simulink model "simpleCylinder1"  (Simulink 6.5)
settings: Solver=ode4  StartTime=0.0  StopTime=inf  FixedStep=0.001  RelTol=1e-3
undefined symbols (not defined in the file or in its folder): x
libraries: dsparch4 x5, xpclib x4, simulink x4
settings Model: Creator=Administrator  LastModifiedBy=PC  BufferReuse=off
settings ConfigSet: SimulationMode=external
settings OptimizationCC: BlockReduction=off  OptimizeBlockIOStorage=off  BufferReuse=off  ExpressionFolding=off  LocalBlockOutputs=off
settings RTWCC: SystemTargetFile=xpctarget.tlc  TemplateMakefile=xpc_default_tmf  Description=xPC Target  ProcessScript=xpctarget_make_rtw_hook
settings xpcTargetCC: TargetFcnLib=ansi_tfl_tmw.mat  GenFloatMathFcnCalls=ANSI_C  ExtModeInterfaceLevel=Level2 - Open

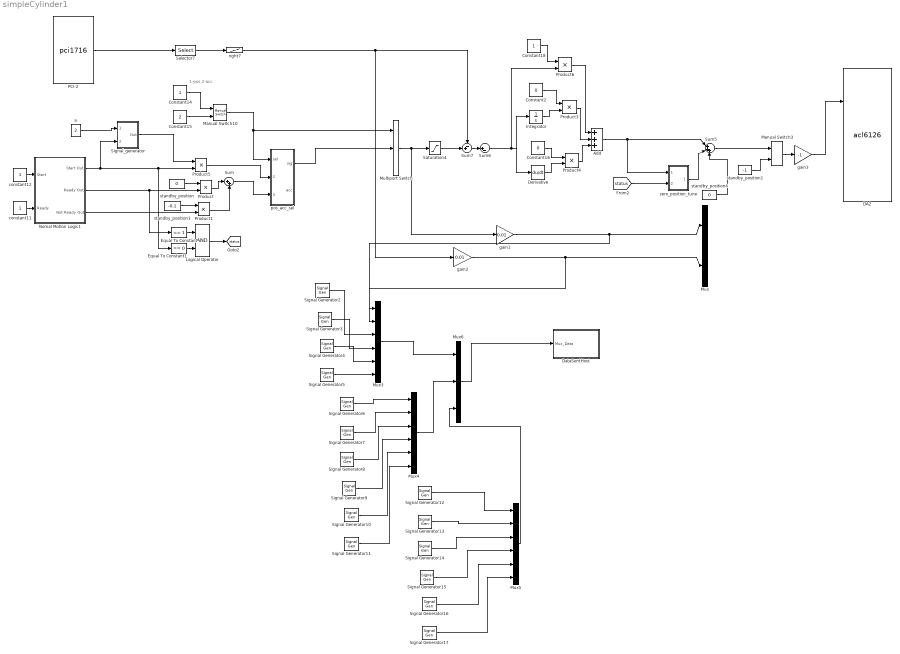
== system simpleCylinder1 ==
  note: 1-pos
      | 2-acc
  Add : Sum  Inputs=+++  OutScaling=2^-10
  Constant14 : Constant  Value=1  OutDataType=fixdt(1,16,0)  ConRadixGroup=Use specified scaling  OutScaling=[]  SampleTime=inf  FramePeriod=inf
  Constant15 : Constant  Value=2  OutDataType=fixdt(1,16,0)  ConRadixGroup=Use specified scaling  OutScaling=[]  SampleTime=inf  FramePeriod=inf
  Constant16 : Constant  Value=0  OutDataType=fixdt(1,16,0)  ConRadixGroup=Use specified scaling  OutScaling=[]  SampleTime=inf  FramePeriod=inf
  Constant18 : Constant  Value=1  OutDataType=fixdt(1,16,0)  ConRadixGroup=Use specified scaling  OutScaling=[]  SampleTime=inf  FramePeriod=inf
  Constant2 : Constant  Value=0  OutDataType=fixdt(1,16,0)  ConRadixGroup=Use specified scaling  OutScaling=[]  SampleTime=inf  FramePeriod=inf
  DA2 : S-Function  FunctionName=acl6126  Parameters=convBaseAddr,Range,[SampleTime SampleOffset]  mask(ACL-6126){sBaseAddr=0x2c0, Ranges=-10, sample=0.001}
      mask prompts: sBaseAddr "Base Address:"; sample "Sample Time:"
      mask help:
      | ACL-6126
      | HIT
      | Analog Output
      mask init:
      | convBaseAddr = 512;Range=10;SampleTime = 0.001; SampleOffset = 0;
      | sampleLength = length (sample);
      | if (sampleLength == 2)
      |   SampleTime = sample(1);
      |   SampleOffset = sample(2);
      | else
      |   SampleTime = sample(1);
      |   SampleOffset = 0;
      | end
      | 
      | sBaseAddr(find(sBaseAddr=='''')) = [];
      | index = findstr(lower(sBaseAddr),'0x');
      | if ~isempty(index) & index==1
      |   BaseAddr = sBaseAddr(3:end);
      |   baLength = length (BaseAddr);
      |   baseStringMember = [abs('0'):abs('9'),abs('a'):abs('f'),abs('A'):abs('F')];
      |   for i = 1:baLength
      |  %   if ~ismember(BaseAddr(i),baseStringMember)
      |  %     error ('Invalid character in hexadecimal string');
      |  %   end
      |   end
      |   convBaseAddr = hex2dec(BaseAddr);
      | else
      |   convBaseAddr = str2num(BaseAddr);
      |   end
      |  Range=Ranges;
      mask Help: helpview([docroot '/toolbox/xpc/pt_io_block_reference.html#xpcioref'])
      mask Display:
      | disp('ACL-6126\ncumt\nAnalog Output');
      | port_label('input',1 , '1');
      | port_label('input',2 , '2');
      | port_label('input',3 , '3');
      | port_label('input',4 , '4');
      | port_label('input',5, '5');
      | port_label('input',6 , '6');
  DataSentHost : Subsystem
  Derivative : Derivative
  Equal To Constant : simulink/Logic and Bit Operations/Compare To Constant  SystemSampleTime=-1  relop===  const=1  LogicOutDataTypeMode=uint8  ZeroCross=off
  Equal To Constant1 : simulink/Logic and Bit Operations/Compare To Constant  SystemSampleTime=-1  relop===  const=0  LogicOutDataTypeMode=uint8  ZeroCross=off
  Integrator : Integrator
  Logical Operator : Logic  AllPortsSameDT=off
  Manual Switch10 : simulink/Signal Routing/Manual Switch  SystemSampleTime=-1  sw=1  action=0
  Manual Switch3 : simulink/Signal Routing/Manual Switch  SystemSampleTime=-1  sw=0  action=0
  Multiport Switch : MultiPortSwitch  Inputs=2  SaturateOnIntegerOverflow=on
  Mux : Mux  Inputs=2
  Mux3 : Mux  Inputs=6
  Mux4 : Mux  Inputs=6
  Mux5 : Mux  Inputs=6
  Mux6 : Mux  Inputs=3
  Nomal Motion Logic1 : Subsystem  AncestorBlock=control_logic_lib/Control Logic(Stateflow Chart)
  PCI-2 : S-Function  FunctionName=pci1716  Parameters=[SampleTime SampleOffset], SLOT  mask(hitad3){Sample=0.001, SLOT=-1}
      mask prompts: Sample "Sample Time:"
      mask help:
      | PCi1716
      | A/D Card
      | Developed by ZhaoJinsong
      | 2012.06.02
      mask init:
      | SampleTime = 0.001; SampleOffset=0;
      mask Help: helpview([docroot '/toolbox/xpc/pt_io_block_reference.html#xpcioref'])
      mask Display:
      | disp('PCI1716  ');
      | 
      | port_label('output',1 , 'OUT');
  Product : Product  OutDataType=fixdt(1,16,0)  OutScaling=[]  SaturateOnIntegerOverflow=on
  Product1 : Product  OutDataType=fixdt(1,16,0)  OutScaling=[]  SaturateOnIntegerOverflow=on
  Product3 : Product  RndMeth=Zero
  Product4 : Product  RndMeth=Zero
  Product5 : Product  OutDataType=fixdt(1,16,0)  OutScaling=[]  SaturateOnIntegerOverflow=on
  Product6 : Product  RndMeth=Zero
  Saturation4 : Saturate  UpperLimit=10  LowerLimit=-10
  Selector7 : Selector  InputType=Vector  ElementSrc=Internal  Elements=2  RowSrc=Internal  Rows=1  ColumnSrc=Internal  Columns=1  IndexIsStartValue=off
  Signal Generator10 : SignalGenerator  Amplitude=11  Frequency=10
  Signal Generator11 : SignalGenerator  Amplitude=12  Frequency=10
  Signal Generator12 : SignalGenerator  Amplitude=13  Frequency=10
  Signal Generator13 : SignalGenerator  Amplitude=14  Frequency=10
  Signal Generator14 : SignalGenerator  Amplitude=15  Frequency=10
  Signal Generator15 : SignalGenerator  Amplitude=16  Frequency=10
  Signal Generator16 : SignalGenerator  Amplitude=17  Frequency=10
  Signal Generator17 : SignalGenerator  Amplitude=18  Frequency=10
  Signal Generator2 : SignalGenerator  Amplitude=3  Frequency=10
  Signal Generator3 : SignalGenerator  Amplitude=4  Frequency=10
  Signal Generator4 : SignalGenerator  Amplitude=5  Frequency=10
  Signal Generator5 : SignalGenerator  Amplitude=6  Frequency=10
  Signal Generator6 : SignalGenerator  Amplitude=7  Frequency=10
  Signal Generator7 : SignalGenerator  Amplitude=8  Frequency=10
  Signal Generator8 : SignalGenerator  Amplitude=9  Frequency=10
  Signal Generator9 : SignalGenerator  Amplitude=10  Frequency=10
  Signal_generator : Subsystem
  Sum : Sum  Inputs=|++  OutDataType=fixdt(1,16,0)  OutScaling=[]  SaturateOnIntegerOverflow=on
  Sum5 : Sum  Inputs=|+++  OutDataType=fixdt(1,16,0)  OutScaling=[]  SaturateOnIntegerOverflow=on
  Sum6 : Sum  Inputs=|+-  OutDataType=fixdt(1,16,0)  OutScaling=[]  SaturateOnIntegerOverflow=on
  Sum7 : Sum  Inputs=-+|  OutDataType=fixdt(1,16,0)  OutScaling=[]  SaturateOnIntegerOverflow=on
  a : Constant  Value=2  OutDataType=fixdt(1,16,0)  ConRadixGroup=Use specified scaling  OutScaling=[]  SampleTime=inf  FramePeriod=inf
  constant11 : Constant  Value=1  OutDataType=sfix(16)  ConRadixGroup=Use specified scaling  OutScaling=2^0  SampleTime=inf  FramePeriod=inf
      settings: OpenFcn=|
      | if get_param(gcb,'value')=='1',
      | set_param(gcb,'value','0');
      | else
      | set_param(gcb,'value','1');end
  constant12 : Constant  Value=1  OutDataType=sfix(16)  ConRadixGroup=Use specified scaling  OutScaling=2^0  SampleTime=inf  FramePeriod=inf
      settings: OpenFcn=|
      | if get_param(gcb,'value')=='1',
      | set_param(gcb,'value','0');
      | else
      | set_param(gcb,'value','1');end
  gain1 : Gain  Gain=0.01  ParameterDataType=fixdt(1,16,0)  ParameterScaling=[]  OutDataType=fixdt(1,16,0)  OutScaling=[]  SaturateOnIntegerOverflow=on
  gain2 : Gain  Gain=0.01  ParameterDataType=fixdt(1,16,0)  ParameterScaling=[]  OutDataType=fixdt(1,16,0)  OutScaling=[]  SaturateOnIntegerOverflow=on
  gain3 : Gain  Gain=-1  ParameterDataType=fixdt(1,16,0)  ParameterScaling=[]  OutDataType=fixdt(1,16,0)  OutScaling=[]  SaturateOnIntegerOverflow=on
  pos_acc_sel : Subsystem
  right7 : Lookup  InputValues=[-0.28 9.725]  OutputValues=[-10 10]  LookUpMeth=Interpolation-Extrapolation  OutDataType=fixdt(1,16,0)  OutScaling=[]  SaturateOnIntegerOverflow=on  SampleTime=-1  LUTDesignTableMode=Redesign Table  LUTDesignDataSource=Block Dialog  LUTDesignFunctionName=sqrt(x)  LUTDesignUseExistingBP=on  LUTDesignRelError=0.01  LUTDesignAbsError=1e-6  RndMeth=Floor
      settings: LockScale=off
  standby_position : Constant  Value=0  OutDataType=fixdt(1,16,0)  ConRadixGroup=Use specified scaling  OutScaling=[]  SampleTime=inf  FramePeriod=inf
  standby_position1 : Constant  Value=-1  OutDataType=fixdt(1,16,0)  ConRadixGroup=Use specified scaling  OutScaling=[]  SampleTime=inf  FramePeriod=inf
  standby_position3 : Constant  Value=-0.1  OutDataType=fixdt(1,16,0)  ConRadixGroup=Use specified scaling  OutScaling=[]  SampleTime=inf  FramePeriod=inf
  standby_position4 : Constant  Value=0  OutDataType=fixdt(1,16,0)  ConRadixGroup=Use specified scaling  OutScaling=[]  SampleTime=inf  FramePeriod=inf
  zero_position_tune : Subsystem
  tag scope: status=global
  wires:
  standby_position1/1 -> Manual Switch3/2
  Manual Switch3/1 -> gain3/1
  Mux5/1 -> Mux6/3
  Mux4/1 -> Mux6/2
  Signal Generator12/1 -> Mux5/1
  Signal Generator13/1 -> Mux5/2
  Signal Generator14/1 -> Mux5/3
  Signal Generator15/1 -> Mux5/4
  Signal Generator16/1 -> Mux5/5
  Signal Generator17/1 -> Mux5/6
  Signal Generator6/1 -> Mux4/1
  Signal Generator7/1 -> Mux4/2
  Signal Generator8/1 -> Mux4/3
  Signal Generator9/1 -> Mux4/4
  Signal Generator10/1 -> Mux4/5
  Signal Generator11/1 -> Mux4/6
  Signal Generator5/1 -> Mux3/6
  Sum5/1 -> Manual Switch3/1
  standby_position4/1 -> Sum5/3
  Sum6/1 -> Product6/2, Integrator/1, Derivative/1
  Sum7/1 -> Sum6/1
  Multiport Switch/1 -> gain1/1, Saturation4/1
  pos_acc_sel/1(sig) -> Multiport Switch/2
  Saturation4/1 -> Sum7/2
  [status] -> zero_position_tune/2(status)
  zero_position_tune/1(Out) -> Sum5/2
  Constant2/1 -> Product3/1
  Integrator/1 -> Product3/2
  Constant16/1 -> Product4/1
  Derivative/1 -> Product4/2
  Constant18/1 -> Product6/1
  Product6/1 -> Add/1
  Product3/1 -> Add/2
  Product4/1 -> Add/3
  Add/1 -> Sum5/1, zero_position_tune/1(error_in)
  gain1/1 -> Mux/1, Mux3/1
  gain2/1 -> Mux/2, Mux3/2
  Mux6/1 -> DataSentHost/1(Mux_Data)
  Mux3/1 -> Mux6/1
  Signal Generator2/1 -> Mux3/3
  Signal Generator3/1 -> Mux3/4
  Signal Generator4/1 -> Mux3/5
  PCI-2/1 -> Selector7/1
  Selector7/1 -> right7/1
  right7/1 -> Sum7/1, gain2/1
  constant12/1 -> Nomal Motion Logic1/1(Start)
  Nomal Motion Logic1/2(Ready Out) -> Product/2, Equal To Constant/1
  standby_position/1 -> Product/1
  Product/1 -> Sum/1
  Sum/1 -> pos_acc_sel/3(ini_pos)
  Nomal Motion Logic1/1(Start Out) -> Product5/2, Equal To Constant1/1, Signal_generator/2(start)
  Product5/1 -> pos_acc_sel/2(sig_in)
  standby_position3/1 -> Product1/1
  Product1/1 -> Sum/2
  Manual Switch10/1 -> Multiport Switch/1, pos_acc_sel/1(sel)
  Constant14/1 -> Manual Switch10/1
  Constant15/1 -> Manual Switch10/2
  Nomal Motion Logic1/3(Not Ready Out) -> Product1/2
  Equal To Constant/1 -> Logical Operator/1
  Equal To Constant1/1 -> Logical Operator/2
  Logical Operator/1 -> [status]
  constant11/1 -> Nomal Motion Logic1/2(Ready)
  Signal_generator/1(Out) -> Product5/1
  a/1 -> Signal_generator/1(sig_sel)
  gain3/1 -> DA2/2

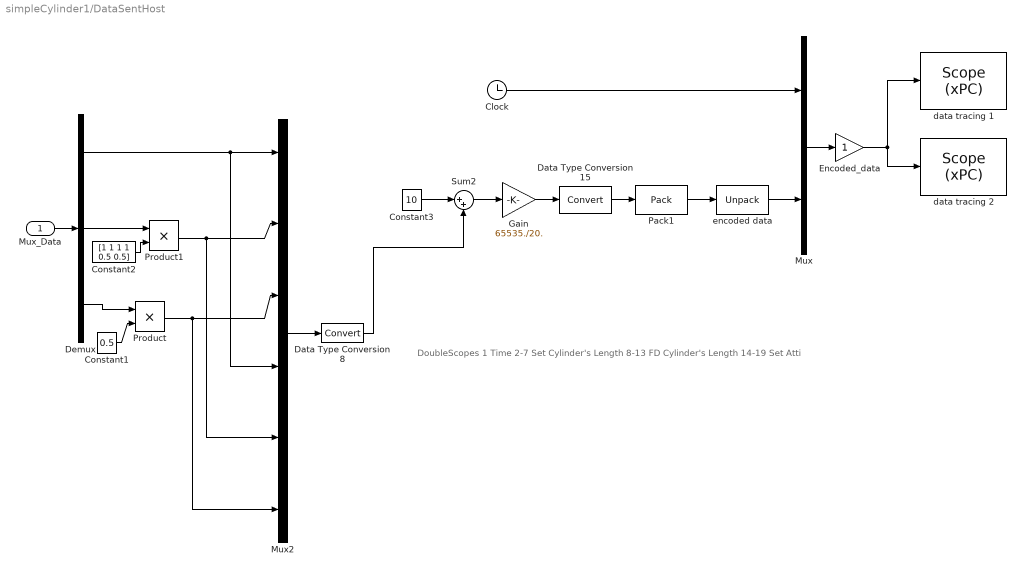
== system simpleCylinder1/DataSentHost ==
  note: DoubleScopes
      | 1          Time
      | 2-7       Set Cylinder's Length
      | 8-13     FD Cylinder's Length
      | 14-19   Set Atti
  Mux_Data : Inport
  Clock : Clock
      settings: Decimation=10
  Constant1 : Constant  Value=0.5  OutDataType=sfix(16)  ConRadixGroup=Use specified scaling  OutScaling=2^0  SampleTime=inf  FramePeriod=inf
  Constant2 : Constant  Value=[1 1 1 1 0.5 0.5]  OutDataType=sfix(16)  ConRadixGroup=Use specified scaling  OutScaling=2^0  SampleTime=inf  FramePeriod=inf
  Constant3 : Constant  Value=10  OutDataType=sfix(16)  ConRadixGroup=Use specified scaling  OutScaling=2^0  SampleTime=inf  FramePeriod=inf
  Data Type Conversion15 : DataTypeConversion  OutDataTypeMode=uint16  SaturateOnIntegerOverflow=on  RndMeth=Zero
  Data Type Conversion8 : DataTypeConversion  OutDataTypeMode=double  SaturateOnIntegerOverflow=on  RndMeth=Zero
  Demux : Demux  Outputs=3
  Encoded_data : Gain
  Gain : Gain  Gain=65535./20.  RndMeth=Nearest  SaturateOnIntegerOverflow=on
  Mux : Mux  Inputs=2
  Mux2 : Mux  Inputs=6
  Pack1 : xpclib/UDP/Pack  datatypes={'uint16'}  byteAlign=1
  Product : Product  RndMeth=Zero
  Product1 : Product  RndMeth=Zero
  Sum2 : Sum  Inputs=|++  SaturateOnIntegerOverflow=on
  data tracing 1 : xpclib/Misc./Scope (xPC)   SystemSampleTime=-1  scopeno=5  scopetype=Host  autostart=off  viewmode=Graphical redraw  formatstr='%15.6f'  grid=on  ylimits=[0,0]  nosamples=500  noprepostsamples=0  interleave=1  triggermode=Scope triggering  triggersignal=1  triggerlevel=0.0  triggerslope=Either  triggerscope=5  triggersample=-1  filename=data.dat  mode=Lazy  writesize=512  autorestart=off
  data tracing 2 : xpclib/Misc./Scope (xPC)   SystemSampleTime=-1  scopeno=4  scopetype=Host  autostart=off  viewmode=Graphical redraw  formatstr='%15.6f'  grid=on  ylimits=[0,0]  nosamples=500  noprepostsamples=0  interleave=1  triggermode=Scope triggering  triggersignal=1  triggerlevel=0.0  triggerslope=Either  triggerscope=4  triggersample=-1  filename=data.dat  mode=Lazy  writesize=512  autorestart=off
  encoded data : xpclib/UDP/Unpack  dimensions={[9]}  datatypes={'double'}  byteAlign=1
  wires:
  Constant2/1 -> Product1/2
  Product1/1 -> Mux2/5, Mux2/2
  Demux/2 -> Product1/1
  Product/1 -> Mux2/6, Mux2/3
  Constant1/1 -> Product/2
  Demux/3 -> Product/1
  Encoded_data/1 -> data tracing 2/1, data tracing 1/1
  Mux/1 -> Encoded_data/1
  Demux/1 -> Mux2/4, Mux2/1
  Mux_Data/1 -> Demux/1
  Clock/1 -> Mux/1
  Constant3/1 -> Sum2/1
  Sum2/1 -> Gain/1
  Pack1/1 -> encoded data/1
  Gain/1 -> Data Type Conversion15/1
  Data Type Conversion15/1 -> Pack1/1
  encoded data/1 -> Mux/2
  Mux2/1 -> Data Type Conversion8/1
  Data Type Conversion8/1 -> Sum2/2

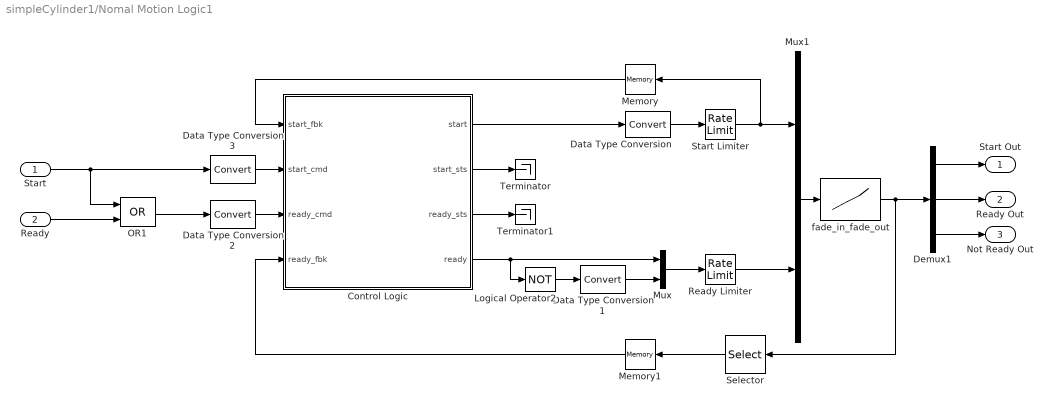
== system simpleCylinder1/Nomal Motion Logic1 ==
  Start : Inport
  Ready : Inport  Port=2
  Control Logic : Stateflow chart
  Data Type Conversion{,1..3} (4 alike) : DataTypeConversion  OutDataTypeMode=double  SaturateOnIntegerOverflow=on  RndMeth=Zero
  Demux1 : Demux  Outputs=3
  Logical Operator2 : Logic  Operator=NOT  Inputs=3  AllPortsSameDT=off
  Memory : Memory  Orientation=left
  Memory1 : Memory  Orientation=left
  Mux : Mux  Inputs=2
  Mux1 : Mux  Inputs=2
  OR1 : Logic  Operator=OR  AllPortsSameDT=off
  Ready Limiter : RateLimiter  RisingSlewLimit=1/5  FallingSlewLimit=-1/5
  Selector : Selector  Orientation=left  InputType=Vector  ElementSrc=Internal  Elements=[2]  RowSrc=Internal  Rows=[2]  ColumnSrc=Internal  Columns=1  InputPortWidth=3  IndexIsStartValue=off  OutputPortSize=[(-2)]
  Start Limiter : RateLimiter  RisingSlewLimit=1/3  FallingSlewLimit=-1/3
  Terminator : Terminator
  Terminator1 : Terminator
  fade_in_fade_out : Lookup  InputValues=[0:0.001:1]  OutputValues=(sin(([0:0.001:1]*2-1)*pi/2)+1)/2  LookUpMeth=Interpolation-Extrapolation  OutDataType=sfix(16)  OutScaling=2^0  SaturateOnIntegerOverflow=on  SampleTime=-1  LUTDesignTableMode=Redesign Table  LUTDesignDataSource=Block Dialog  LUTDesignFunctionName=sqrt(x)  LUTDesignUseExistingBP=on  LUTDesignRelError=0.01  LUTDesignAbsError=1e-6  RndMeth=Floor
      settings: LockScale=off
  Start Out : Outport
  Ready Out : Outport  Port=2
  Not Ready Out : Outport  Port=3
  wires:
  Ready/1 -> OR1/2
  Start/1 -> OR1/1, Data Type Conversion3/1
  Control Logic/3(ready_sts) -> Terminator1/1
  Control Logic/2(start_sts) -> Terminator/1
  OR1/1 -> Data Type Conversion2/1
  Data Type Conversion3/1 -> Control Logic/2(start_cmd)
  Demux1/3 -> Not Ready Out/1
  Demux1/1 -> Start Out/1
  Demux1/2 -> Ready Out/1
  Data Type Conversion/1 -> Start Limiter/1
  Start Limiter/1 -> Mux1/1, Memory/1
  Control Logic/1(start) -> Data Type Conversion/1
  Control Logic/4(ready) -> Logical Operator2/1, Mux/1
  Logical Operator2/1 -> Data Type Conversion1/1
  Mux/1 -> Ready Limiter/1
  Ready Limiter/1 -> Mux1/2
  Mux1/1 -> fade_in_fade_out/1
  fade_in_fade_out/1 -> Selector/1, Demux1/1
  Memory/1 -> Control Logic/1(start_fbk)
  Memory1/1 -> Control Logic/4(ready_fbk)
  Data Type Conversion1/1 -> Mux/2
  Data Type Conversion2/1 -> Control Logic/3(ready_cmd)
  Selector/1 -> Memory1/1

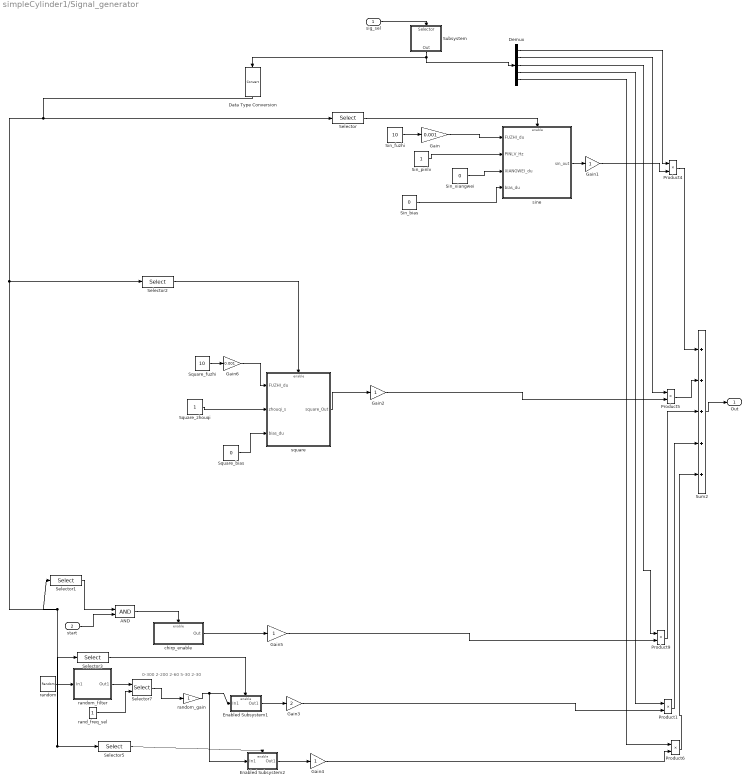
== system simpleCylinder1/Signal_generator ==
  note: 0-300
      | 2-200
      | 2-60
      | 5-30
      | 2-30
  sig_sel : Inport  OutDataType=fixdt(1,16,0)  OutScaling=[]
  start : Inport  Port=2  OutDataType=fixdt(1,16,0)  OutScaling=[]
  AND : Logic  AllPortsSameDT=off  OutDataTypeMode=Specify via dialog
  Data Type Conversion : DataTypeConversion  Orientation=down  OutDataTypeMode=boolean  OutDataType=fixdt(1,16,0)  OutScaling=[]  SaturateOnIntegerOverflow=on  RndMeth=Zero
  Demux : Demux  Outputs=5
  Enabled Subsystem1 : Subsystem  TreatAsAtomicUnit=on
  Enabled Subsystem2 : Subsystem  TreatAsAtomicUnit=on
  Gain : Gain  Gain=0.001
  Gain{1..2,4..5} (4 alike) : Gain  ParameterDataType=fixdt(1,16,0)  ParameterScaling=[]  OutDataType=fixdt(1,16,0)  OutScaling=[]  SaturateOnIntegerOverflow=on
  Gain3 : Gain  Gain=2  ParameterDataType=fixdt(1,16,0)  ParameterScaling=[]  OutDataType=fixdt(1,16,0)  OutScaling=[]  SaturateOnIntegerOverflow=on
  Gain6 : Gain  Gain=0.001
  Product{1,4..6,9} (5 alike) : Product  OutDataType=fixdt(1,16,0)  OutScaling=[]  SaturateOnIntegerOverflow=on
  Selector : Selector  InputType=Vector  ElementSrc=Internal  Elements=1  RowSrc=Internal  Rows=2  ColumnSrc=Internal  Columns=1  InputPortWidth=5  IndexIsStartValue=off  OutputPortSize=[(-2)]
  Selector1 : Selector  InputType=Vector  ElementSrc=Internal  Elements=3  RowSrc=Internal  Rows=4  ColumnSrc=Internal  Columns=1  InputPortWidth=5  IndexIsStartValue=off  OutputPortSize=[(-2)]
  Selector2 : Selector  InputType=Vector  ElementSrc=Internal  Elements=2  RowSrc=Internal  Rows=3  ColumnSrc=Internal  Columns=1  InputPortWidth=5  IndexIsStartValue=off  OutputPortSize=[(-2)]
  Selector3 : Selector  InputType=Vector  ElementSrc=Internal  Elements=4  RowSrc=Internal  Rows=5  ColumnSrc=Internal  Columns=1  InputPortWidth=5  IndexIsStartValue=off  OutputPortSize=[(-2)]
  Selector5 : Selector  InputType=Vector  ElementSrc=Internal  Elements=5  RowSrc=Internal  Rows=6  ColumnSrc=Internal  Columns=1  InputPortWidth=5  IndexIsStartValue=off  OutputPortSize=[(-2)]
  Selector7 : Selector  InputType=Vector  ElementSrc=External  Elements=[1 3]  RowSrc=External  Rows=[1 3]  ColumnSrc=Internal  Columns=1  InputPortWidth=5  IndexIsStartValue=off  OutputPortSize=[(-2)]
  Sin_bias : Constant  Value=0  OutDataType=sfix(16)  ConRadixGroup=Use specified scaling  OutScaling=2^0  SampleTime=inf  FramePeriod=inf
  Sin_fuzhi : Constant  Value=10  OutDataType=sfix(16)  ConRadixGroup=Use specified scaling  OutScaling=2^0  SampleTime=inf  FramePeriod=inf
  Sin_pinlv : Constant  Value=1  OutDataType=sfix(16)  ConRadixGroup=Use specified scaling  OutScaling=2^0  SampleTime=inf  FramePeriod=inf
  Sin_xiangwei : Constant  Value=0  OutDataType=sfix(16)  ConRadixGroup=Use specified scaling  OutScaling=2^0  SampleTime=inf  FramePeriod=inf
  Square_bias : Constant  Value=0  OutDataType=sfix(16)  ConRadixGroup=Use specified scaling  OutScaling=2^0  SampleTime=inf  FramePeriod=inf
  Square_fuzhi : Constant  Value=10  OutDataType=sfix(16)  ConRadixGroup=Use specified scaling  OutScaling=2^0  SampleTime=inf  FramePeriod=inf
  Square_zhouqi : Constant  Value=1  OutDataType=sfix(16)  ConRadixGroup=Use specified scaling  OutScaling=2^0  SampleTime=inf  FramePeriod=inf
  Subsystem : Subsystem  Orientation=down  mask{itnum=5}
      mask prompts: itnum "Signals Number"
  Sum2 : Sum  Inputs=+++++  OutDataType=fixdt(1,16,0)  OutScaling=[]  SaturateOnIntegerOverflow=on
  chirp_enable : Subsystem  TreatAsAtomicUnit=on
  rand_freq_sel : Constant  Value=1  OutDataType=fixdt(1,16,0)  ConRadixGroup=Use specified scaling  OutScaling=[]  SampleTime=inf  FramePeriod=inf
  random : UniformRandomNumber  SampleTime=0
  random_filter : Subsystem
  random_gain : Gain  ParameterDataType=fixdt(1,16,0)  ParameterScaling=[]  OutDataType=fixdt(1,16,0)  OutScaling=[]  SaturateOnIntegerOverflow=on
  sine : Subsystem
  square : Subsystem
  Out : Outport  OutDataType=fixdt(1,16,0)  OutScaling=[]
  wires:
  Product6/1 -> Sum2/5
  Demux/5 -> Product6/1
  Demux/4 -> Product1/1
  Gain5/1 -> Product9/2
  Demux/3 -> Product9/1
  Gain2/1 -> Product5/2
  Demux/2 -> Product5/1
  Product4/1 -> Sum2/1
  Demux/1 -> Product4/1
  Square_bias/1 -> square/3(bias_du)
  Sin_bias/1 -> sine/4(bias_du)
  Square_zhouqi/1 -> square/2(zhouqi_s)
  Square_fuzhi/1 -> Gain6/1
  Sin_xiangwei/1 -> sine/3(XIANGWEI_du)
  Sin_fuzhi/1 -> Gain/1
  Sin_pinlv/1 -> sine/2(PINLV_Hz)
  Selector/1 -> sine/Enable
  Gain3/1 -> Product1/2
  Product1/1 -> Sum2/4
  Selector7/1 -> random_gain/1
  Gain4/1 -> Product6/2
  Enabled Subsystem1/1(Out1) -> Gain3/1
  random_gain/1 -> Enabled Subsystem2/1(In1), Enabled Subsystem1/1(In1)
  Selector3/1 -> Enabled Subsystem1/Enable
  rand_freq_sel/1 -> Selector7/2
  random_filter/1(Out1) -> Selector7/1
  random/1 -> random_filter/1(In1)
  chirp_enable/1(Out) -> Gain5/1
  start/1 -> AND/2
  Selector1/1 -> AND/1
  AND/1 -> chirp_enable/Enable
  Enabled Subsystem2/1(Out1) -> Gain4/1
  sine/1(sin_out) -> Gain1/1
  Selector5/1 -> Enabled Subsystem2/Enable
  Selector2/1 -> square/Enable
  square/1(square_Out) -> Gain2/1
  Data Type Conversion/1 -> Selector/1, Selector3/1, Selector5/1, Selector1/1, Selector2/1
  Sum2/1 -> Out/1
  Product5/1 -> Sum2/2
  Product9/1 -> Sum2/3
  Subsystem/1(Out) -> Data Type Conversion/1, Demux/1
  sig_sel/1 -> Subsystem/1(Selector)
  Gain1/1 -> Product4/2
  Gain/1 -> sine/1(FUZHI_du)
  Gain6/1 -> square/1(FUZHI_du)

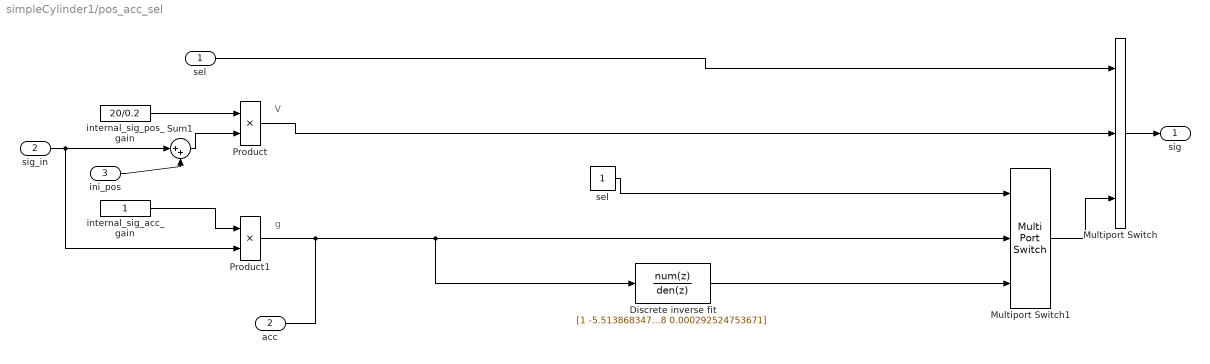
== system simpleCylinder1/pos_acc_sel ==
  note: g
  note: V
  sel : Inport  OutDataType=fixdt(1,16,0)  OutScaling=[]
  sig_in : Inport  Port=2  OutDataType=fixdt(1,16,0)  OutScaling=[]
  ini_pos : Inport  Port=3  OutDataType=fixdt(1,16,0)  OutScaling=[]
  Discrete inverse fit : DiscreteTransferFcn  Numerator=[1 -5.513868347662695 12.88491366007906 -16.323990002559352 11.821537968329908 -4.639485908156727 0.77101716333547]  Denominator=[0.013392688630559 -0.043519228995354 0.057088791124972 -0.038794303856191 0.015270049598488 -0.003637012524308 0.000292524753671]  SampleTime=0.001
  Multiport Switch : MultiPortSwitch  Inputs=2  SaturateOnIntegerOverflow=on
  Multiport Switch1 : MultiPortSwitch  Inputs=2  SaturateOnIntegerOverflow=on
  Product : Product  OutDataType=fixdt(1,16,0)  OutScaling=[]  SaturateOnIntegerOverflow=on
  Product1 : Product  OutDataType=fixdt(1,16,0)  OutScaling=[]  SaturateOnIntegerOverflow=on
  Sum1 : Sum  Inputs=|++  OutDataType=fixdt(1,16,0)  OutScaling=[]  SaturateOnIntegerOverflow=on
  internal_sig_acc_gain : Constant  Value=1  OutDataType=fixdt(1,16,0)  ConRadixGroup=Use specified scaling  OutScaling=[]  SampleTime=inf  FramePeriod=inf
  internal_sig_pos_gain : Constant  Value=20/0.2  OutDataType=fixdt(1,16,0)  ConRadixGroup=Use specified scaling  OutScaling=[]  SampleTime=inf  FramePeriod=inf
  "sel " : Constant  Value=1  OutDataType=fixdt(1,16,0)  ConRadixGroup=Use specified scaling  OutScaling=[]  SampleTime=inf  FramePeriod=inf
  sig : Outport  OutDataType=fixdt(1,16,0)  OutScaling=[]
  acc : Outport  Port=2  OutDataType=fixdt(1,16,0)  OutScaling=[]
  wires:
  internal_sig_acc_gain/1 -> Product1/1
  Product1/1 -> Discrete inverse fit/1, Multiport Switch1/2, acc/1
  internal_sig_pos_gain/1 -> Product/1
  Product/1 -> Multiport Switch/2
  Sum1/1 -> Product/2
  ini_pos/1 -> Sum1/2
  Multiport Switch/1 -> sig/1
  sel/1 -> Multiport Switch/1
  sig_in/1 -> Product1/2, Sum1/1
  Discrete inverse fit/1 -> Multiport Switch1/3
  "sel "/1 -> Multiport Switch1/1
  Multiport Switch1/1 -> Multiport Switch/3

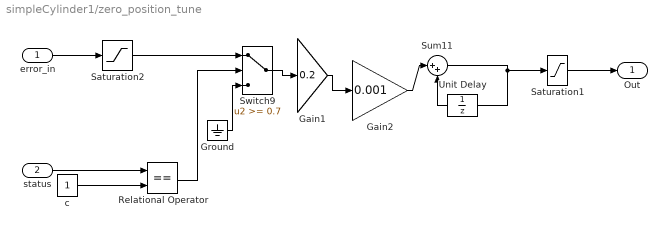
== system simpleCylinder1/zero_position_tune ==
  error_in : Inport  OutDataType=fixdt(1,16,0)  OutScaling=[]
  status : Inport  Port=2  OutDataType=fixdt(1,16,0)  OutScaling=[]
  Gain1 : Gain  Gain=0.2  ParameterDataType=fixdt(1,16,0)  ParameterScaling=[]  OutDataType=fixdt(1,16,0)  OutScaling=[]  SaturateOnIntegerOverflow=on
  Gain2 : Gain  Gain=0.001  ParameterDataType=fixdt(1,16,0)  ParameterScaling=[]  OutDataType=fixdt(1,16,0)  OutScaling=[]  SaturateOnIntegerOverflow=on
  Ground : Ground
  Relational Operator : RelationalOperator  Operator===  InputSameDT=on
  Saturation1 : Saturate
  Saturation2 : Saturate  UpperLimit=0.1  LowerLimit=-0.1
  Sum11 : Sum  Inputs=|++  OutDataType=fixdt(1,16,0)  OutScaling=[]  SaturateOnIntegerOverflow=on  InputSameDT=on
  Switch9 : Switch  Threshold=0.7  SaturateOnIntegerOverflow=on  InputSameDT=on
  Unit Delay : UnitDelay  X0=-0.03  SampleTime=0.001
  c : Constant  Value=1  OutDataTypeMode=boolean  OutDataType=fixdt(1,16,0)  ConRadixGroup=Use specified scaling  OutScaling=[]  SampleTime=inf  FramePeriod=inf
  Out : Outport  OutDataType=fixdt(1,16,0)  OutScaling=[]
  wires:
  Saturation1/1 -> Out/1
  Gain1/1 -> Gain2/1
  status/1 -> Relational Operator/1
  error_in/1 -> Saturation2/1
  Relational Operator/1 -> Switch9/2
  c/1 -> Relational Operator/2
  Saturation2/1 -> Switch9/1
  Ground/1 -> Switch9/3
  Switch9/1 -> Gain1/1
  Sum11/1 -> Saturation1/1, Unit Delay/1
  Gain2/1 -> Sum11/1
  Unit Delay/1 -> Sum11/2

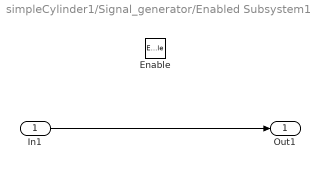
== system simpleCylinder1/Signal_generator/Enabled Subsystem1 ==
  In1 : Inport  OutDataType=fixdt(1,16,0)  OutScaling=[]
  Enable : EnablePort
  Out1 : Outport  OutDataType=fixdt(1,16,0)  OutScaling=[]
  wires:
  In1/1 -> Out1/1

== system simpleCylinder1/Signal_generator/Enabled Subsystem2 ==
  In1 : Inport  OutDataType=fixdt(1,16,0)  OutScaling=[]
  Enable : EnablePort
  Out1 : Outport  OutDataType=fixdt(1,16,0)  OutScaling=[]
  wires:
  In1/1 -> Out1/1

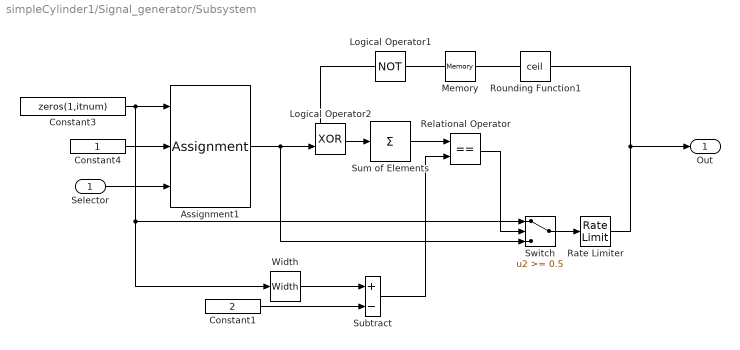
== system simpleCylinder1/Signal_generator/Subsystem ==
  Selector : Inport  OutDataType=fixdt(1,16,0)  OutScaling=[]
  Assignment1 : Assignment  InputType=Vector  IndexIsStartValue=off  ElementSrc=External  Elements=1  RowSrc=External  Rows=1  ColumnSrc=Internal  Columns=1  OutputInitialize=Initialize using input (U1)  OutputDimensions=[([([([([1])])])])]
  Constant1 : Constant  Value=2  OutDataType=fixdt(1,16,0)  ConRadixGroup=Use specified scaling  OutScaling=[]  SampleTime=inf  FramePeriod=inf
  Constant3 : Constant  Value=zeros(1,itnum)  OutDataType=fixdt(1,16,0)  ConRadixGroup=Use specified scaling  OutScaling=[]  SampleTime=inf  FramePeriod=inf
  Constant4 : Constant  Value=1  OutDataType=fixdt(1,16,0)  ConRadixGroup=Use specified scaling  OutScaling=[]  SampleTime=inf  FramePeriod=inf
  Logical Operator1 : Logic  Operator=NOT  AllPortsSameDT=off
  Logical Operator2 : Logic  Operator=XOR  AllPortsSameDT=off
  Memory : Memory  InheritSampleTime=on
  Rate Limiter : RateLimiter  RisingSlewLimit=1/4  FallingSlewLimit=-1/4
  Relational Operator : RelationalOperator  Operator===
  Rounding Function1 : Rounding  Operator=ceil
  Subtract : Sum  Inputs=+-  OutDataTypeMode=double  OutDataType=fixdt(1,16,0)  OutScaling=[]
  Sum of Elements : Sum  Inputs=+  OutDataTypeMode=double  OutDataType=fixdt(1,16,0)  OutScaling=[]
  Switch : Switch  Threshold=0.5  SaturateOnIntegerOverflow=on
  Width : Width
  Out : Outport  OutDataType=fixdt(1,16,0)  OutScaling=[]
  wires:
  Rate Limiter/1 -> Out/1, Rounding Function1/1
  Relational Operator/1 -> Switch/2
  Subtract/1 -> Relational Operator/2
  Sum of Elements/1 -> Relational Operator/1
  Constant1/1 -> Subtract/2
  Width/1 -> Subtract/1
  Logical Operator2/1 -> Sum of Elements/1
  Selector/1 -> Assignment1/3
  Memory/1 -> Logical Operator1/1
  Switch/1 -> Rate Limiter/1
  Logical Operator1/1 -> Logical Operator2/1
  Rounding Function1/1 -> Memory/1
  Assignment1/1 -> Switch/3, Logical Operator2/2
  Constant4/1 -> Assignment1/2
  Constant3/1 -> Switch/1, Width/1, Assignment1/1

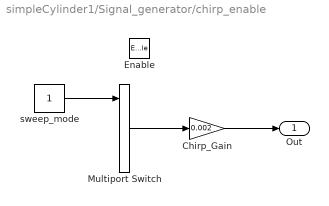
== system simpleCylinder1/Signal_generator/chirp_enable ==
  Enable : EnablePort
  Chirp_Gain : Gain  Gain=0.002  ParameterDataType=fixdt(1,16,0)  ParameterScaling=[]  OutDataType=fixdt(1,16,0)  OutScaling=[]  SaturateOnIntegerOverflow=on
  Multiport Switch : MultiPortSwitch  Inputs=2  SaturateOnIntegerOverflow=on
  sweep_mode : Constant  Value=1  OutDataType=fixdt(1,16,0)  ConRadixGroup=Use specified scaling  OutScaling=[]  SampleTime=inf  FramePeriod=inf
  Out : Outport  OutDataType=fixdt(1,16,0)  OutScaling=[]
  wires:
  Multiport Switch/1 -> Chirp_Gain/1
  sweep_mode/1 -> Multiport Switch/1
  Chirp_Gain/1 -> Out/1

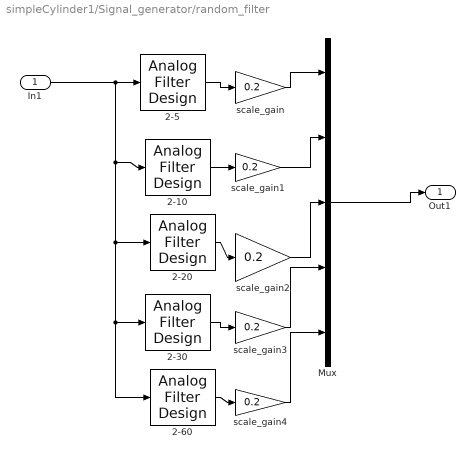
== system simpleCylinder1/Signal_generator/random_filter ==
  In1 : Inport  OutDataType=fixdt(1,16,0)  OutScaling=[]
  2-10 : dsparch4/Analog Filter Design  method=Butterworth  filttype=Bandpass  N=8  Wlo=1*2*pi  Whi=2*2*pi  Rp=2  Rs=40
  2-20 : dsparch4/Analog Filter Design  method=Butterworth  filttype=Bandpass  N=8  Wlo=1*2*pi  Whi=3*2*pi  Rp=2  Rs=40
  2-30 : dsparch4/Analog Filter Design  method=Butterworth  filttype=Bandpass  N=8  Wlo=1*2*pi  Whi=5*2*pi  Rp=2  Rs=40
  2-5 : dsparch4/Analog Filter Design  method=Butterworth  filttype=Bandpass  N=8  Wlo=0.1*2*pi  Whi=1*2*pi  Rp=2  Rs=40
  2-60 : dsparch4/Analog Filter Design  method=Butterworth  filttype=Bandpass  N=8  Wlo=1*2*pi  Whi=10*2*pi  Rp=2  Rs=40
  Mux : Mux  Inputs=5
  scale_gain{,1..4} (5 alike) : Gain  Gain=0.2  ParameterDataType=fixdt(1,16,0)  ParameterScaling=[]  OutDataType=fixdt(1,16,0)  OutScaling=[]  SaturateOnIntegerOverflow=on
  Out1 : Outport  OutDataType=fixdt(1,16,0)  OutScaling=[]
  wires:
  In1/1 -> 2-5/1, 2-60/1, 2-30/1, 2-20/1, 2-10/1
  2-60/1 -> scale_gain4/1
  Mux/1 -> Out1/1
  2-5/1 -> scale_gain/1
  2-10/1 -> scale_gain1/1
  2-20/1 -> scale_gain2/1
  2-30/1 -> scale_gain3/1
  scale_gain/1 -> Mux/1
  scale_gain1/1 -> Mux/2
  scale_gain2/1 -> Mux/3
  scale_gain3/1 -> Mux/4
  scale_gain4/1 -> Mux/5

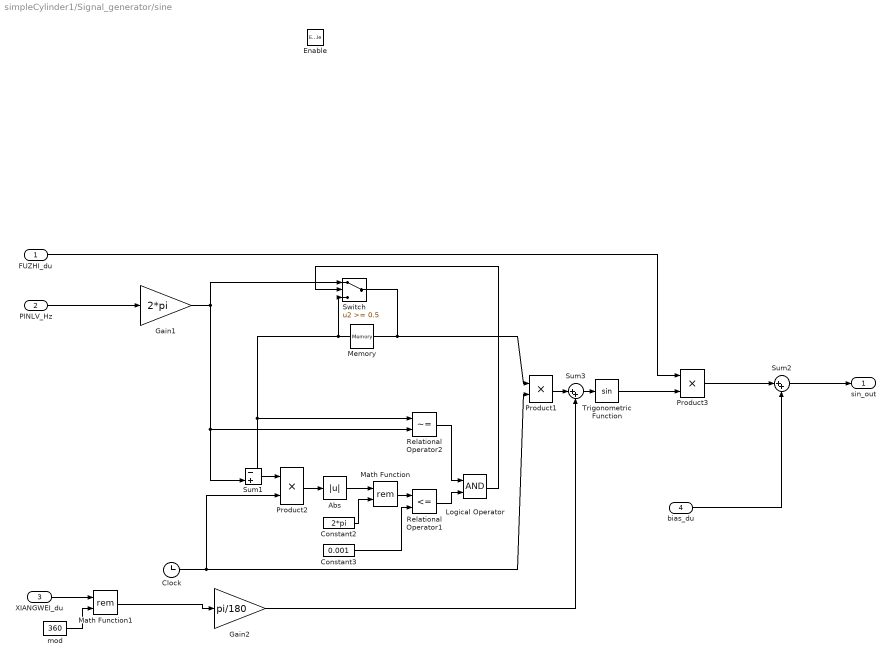
== system simpleCylinder1/Signal_generator/sine ==
  FUZHI_du : Inport  OutDataType=fixdt(1,16,0)  OutScaling=[]
  PINLV_Hz : Inport  Port=2  OutDataType=fixdt(1,16,0)  OutScaling=[]
  XIANGWEI_du : Inport  Port=3  OutDataType=fixdt(1,16,0)  OutScaling=[]
  bias_du : Inport  Port=4  OutDataType=fixdt(1,16,0)  OutScaling=[]
  Enable : EnablePort  StatesWhenEnabling=reset
  Abs : Abs  SaturateOnIntegerOverflow=on  SampleTime=-1
  Clock : Clock
      settings: Decimation=10
  Constant2 : Constant  Value=2*pi  OutDataType=fixdt(1,16,0)  ConRadixGroup=Use specified scaling  OutScaling=[]  SampleTime=inf  FramePeriod=inf
  Constant3 : Constant  Value=0.001  OutDataType=fixdt(1,16,0)  ConRadixGroup=Use specified scaling  OutScaling=[]  SampleTime=inf  FramePeriod=inf
  Gain1 : Gain  Gain=2*pi  ParameterDataType=fixdt(1,16,0)  ParameterScaling=[]  OutDataType=fixdt(1,16,0)  OutScaling=[]  SaturateOnIntegerOverflow=on
  Gain2 : Gain  Gain=pi/180  ParameterDataType=fixdt(1,16,0)  ParameterScaling=[]  OutDataType=fixdt(1,16,0)  OutScaling=[]  SaturateOnIntegerOverflow=on
  Logical Operator : Logic  AllPortsSameDT=off
  Math Function : Math  Operator=rem  OutDataType=fixdt(1,16,0)  OutScaling=[]  SaturateOnIntegerOverflow=on
  Math Function1 : Math  Operator=rem  OutDataType=fixdt(1,16,0)  OutScaling=[]  SaturateOnIntegerOverflow=on
  Memory : Memory
  Product1 : Product  OutDataType=fixdt(1,16,0)  OutScaling=[]  SaturateOnIntegerOverflow=on
  Product2 : Product  OutDataType=fixdt(1,16,0)  OutScaling=[]  SaturateOnIntegerOverflow=on
  Product3 : Product  OutDataType=fixdt(1,16,0)  OutScaling=[]  SaturateOnIntegerOverflow=on
  Relational Operator1 : RelationalOperator  Operator=<=
  Relational Operator2 : RelationalOperator  Operator=~=
  Sum1 : Sum  Inputs=-+  OutDataType=fixdt(1,16,0)  OutScaling=[]  SaturateOnIntegerOverflow=on
  Sum2 : Sum  Inputs=|++  OutDataType=fixdt(1,16,0)  OutScaling=[]  SaturateOnIntegerOverflow=on
  Sum3 : Sum  Inputs=|++  OutDataType=fixdt(1,16,0)  OutScaling=[]  SaturateOnIntegerOverflow=on
  Switch : Switch  Threshold=0.5  SaturateOnIntegerOverflow=on
  Trigonometric Function : Trigonometry
  mod : Constant  Value=360  OutDataType=fixdt(1,16,0)  ConRadixGroup=Use specified scaling  OutScaling=[]  SampleTime=inf  FramePeriod=inf
  sin_out : Outport  OutDataType=fixdt(1,16,0)  OutScaling=[]
  wires:
  Clock/1 -> Product1/2, Product2/2
  Product1/1 -> Sum3/1
  Trigonometric Function/1 -> Product3/2
  Gain2/1 -> Sum3/2
  Sum3/1 -> Trigonometric Function/1
  FUZHI_du/1 -> Product3/1
  Product2/1 -> Abs/1
  Abs/1 -> Math Function/1
  Constant2/1 -> Math Function/2
  Math Function/1 -> Relational Operator1/1
  Constant3/1 -> Relational Operator1/2
  Switch/1 -> Product1/1, Memory/1
  Gain1/1 -> Relational Operator2/2, Sum1/2, Switch/1
  Sum1/1 -> Product2/1
  Relational Operator2/1 -> Logical Operator/1
  Relational Operator1/1 -> Logical Operator/2
  Logical Operator/1 -> Switch/2
  PINLV_Hz/1 -> Gain1/1
  XIANGWEI_du/1 -> Math Function1/1
  Math Function1/1 -> Gain2/1
  mod/1 -> Math Function1/2
  bias_du/1 -> Sum2/2
  Sum2/1 -> sin_out/1
  Product3/1 -> Sum2/1
  Memory/1 -> Sum1/1, Relational Operator2/1, Switch/3

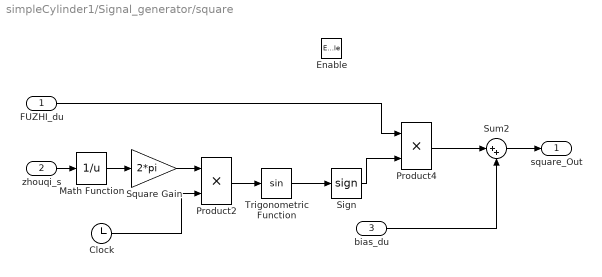
== system simpleCylinder1/Signal_generator/square ==
  FUZHI_du : Inport  OutDataType=fixdt(1,16,0)  OutScaling=[]
  zhouqi_s : Inport  Port=2  OutDataType=fixdt(1,16,0)  OutScaling=[]
  bias_du : Inport  Port=3  OutDataType=fixdt(1,16,0)  OutScaling=[]
  Enable : EnablePort  StatesWhenEnabling=reset
  Clock : Clock
      settings: Decimation=10
  Math Function : Math  Operator=reciprocal  OutDataType=fixdt(1,16,0)  OutScaling=[]  SaturateOnIntegerOverflow=on
  Product2 : Product  OutDataType=fixdt(1,16,0)  OutScaling=[]  SaturateOnIntegerOverflow=on
  Product4 : Product  OutDataType=fixdt(1,16,0)  OutScaling=[]  SaturateOnIntegerOverflow=on
  Sign : Signum
  Square Gain : Gain  Gain=2*pi  ParameterDataType=fixdt(1,16,0)  ParameterScaling=[]  OutDataType=fixdt(1,16,0)  OutScaling=[]  SaturateOnIntegerOverflow=on
  Sum2 : Sum  Inputs=|++  OutDataType=fixdt(1,16,0)  OutScaling=[]  SaturateOnIntegerOverflow=on
  Trigonometric Function : Trigonometry
  square_Out : Outport  OutDataType=fixdt(1,16,0)  OutScaling=[]
  wires:
  Math Function/1 -> Square Gain/1
  Clock/1 -> Product2/2
  Product2/1 -> Trigonometric Function/1
  Trigonometric Function/1 -> Sign/1
  FUZHI_du/1 -> Product4/1
  Sign/1 -> Product4/2
  zhouqi_s/1 -> Math Function/1
  bias_du/1 -> Sum2/2
  Sum2/1 -> square_Out/1
  Product4/1 -> Sum2/1
  Square Gain/1 -> Product2/1

== stateflow chart Nomal Motion Logic1/Control Logic ==
  state run_mode [parallel]
    settings: executionOrder=1
    state running
      du:start=1;start_sts=2;
    state to_stopped
      du:start=0;start_sts=3;
    state to_running
      du:start=1;start_sts=1;
    state stopped
      du:start=0;start_sts=0;
    (default) -> stopped
    stopped -> to_running : [start_cmd&&in(ready_mode.ready)]
    to_running -> running [order 1] : [start_cmd==start_fbk]
    running -> to_stopped : [!start_cmd]
    to_stopped -> stopped [order 2] : [start_cmd==start_fbk]
    to_stopped -> to_running [order 1] : [start_cmd&&in(ready_mode.ready)]
    to_running -> to_stopped [order 2] : [!start_cmd]
  state ready_mode [parallel]
    settings: executionOrder=2
    state ready
      du:ready=1;ready_sts=2;
    state to_rest
      du:ready=0;ready_sts=3;
    state rest
      du:ready=0;ready_sts=0;
    state to_ready
      du:ready=1;ready_sts=1;
    (default) -> rest
    rest -> to_ready : [ready_cmd]
    to_ready -> ready [order 1] : [ready_cmd==ready_fbk]
    ready -> to_rest : [!ready_cmd&&in(run_mode.stopped)]
    to_rest -> rest [order 2] : [ready_cmd==ready_fbk]
    to_rest -> to_ready [order 1] : [ready_cmd]
    to_ready -> to_rest [order 2] : [!ready_cmd&&in(run_mode.stopped)]
  data: start_fbk input double; start_cmd input double; ready_cmd input double; ready_fbk input double; start output boolean; start_sts output double; ready_sts output double; ready output boolean
